simulink model "System_Modell"  (R2018a)
settings: Solver=FixedStepAuto  StartTime=0.0  StopTime=inf  FixedStep=1/f  RelTol=1e-3
values from neighbouring files (symbols this model uses):
  f = 10000    [System_Init.m]
(part 1 of 8)
settings Model: Creator=lenovo  LastModifiedBy=lenovo

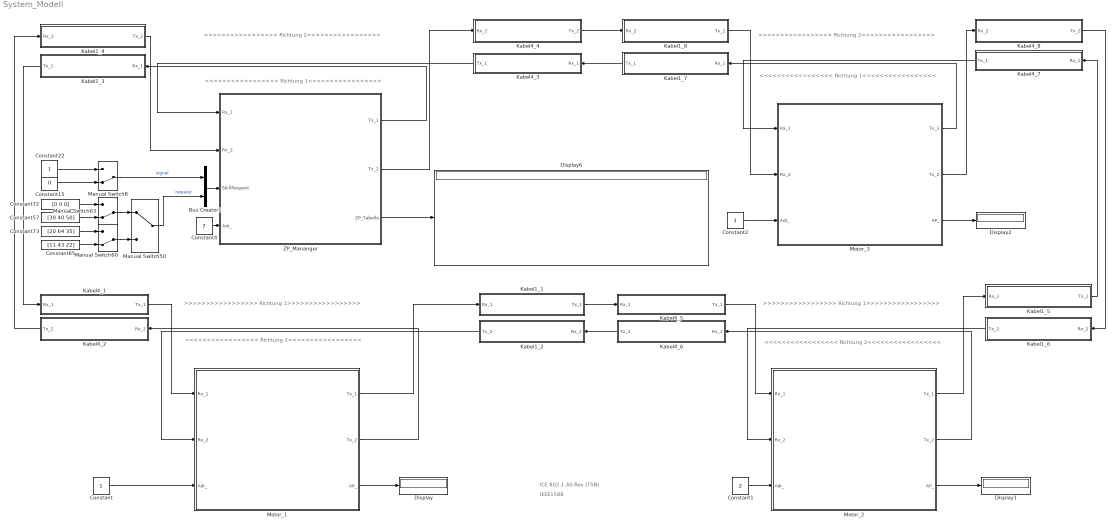
== system System_Modell ==
  note: >>>>>>>>>>>>>>>>> Richtung 1>>>>>>>>>>>>>>>>>
  note: <<<<<<<<<<<<<<<<< Richtung 2<<<<<<<<<<<<<<<<<
  note: ICE 802.1 AS-Rev (TSN)
  note: IEEE1588
  note: >>>>>>>>>>>>>>>>> Richtung 2>>>>>>>>>>>>>>>>>
  note: <<<<<<<<<<<<<<<<< Richtung 1<<<<<<<<<<<<<<<<<
  note: >>>>>>>>>>>>>>>>> Richtung 2>>>>>>>>>>>>>>>>>
  note: <<<<<<<<<<<<<<<<< Richtung 1<<<<<<<<<<<<<<<<<
  note: >>>>>>>>>>>>>>>>> Richtung 1>>>>>>>>>>>>>>>>>
  note: <<<<<<<<<<<<<<<<< Richtung 2<<<<<<<<<<<<<<<<<
  Bus Creator1 : BusCreator  Inputs=2
  Constant : Constant  OutDataTypeStr=double
  Constant1 : Constant  Value=2  OutDataTypeStr=double
  Constant15 : Constant  Value=0  OutDataTypeStr=boolean
  Constant2 : Constant  Value=3  OutDataTypeStr=double
  Constant22 : Constant  OutDataTypeStr=boolean
  Constant4 : Constant  Value=7  OutDataTypeStr=double
  Constant57 : Constant  Value=[30 40 50]
  Constant65 : Constant  Value=[11 43 22]
  Constant72 : Constant  Value=[0 0 0]
  Constant73 : Constant  Value=[20 64 35]
  Display{,1..2,6} (4 alike) : Display
  Kabel1_1 : Subsystem  TreatAsAtomicUnit=on
  Kabel1_2 : Subsystem  TreatAsAtomicUnit=on
  Kabel1_3 : Subsystem  TreatAsAtomicUnit=on
  Kabel1_4 : Subsystem  TreatAsAtomicUnit=on
  Kabel1_5 : Subsystem  TreatAsAtomicUnit=on
  Kabel1_6 : Subsystem  TreatAsAtomicUnit=on
  Kabel1_7 : Subsystem  TreatAsAtomicUnit=on
  Kabel1_8 : Subsystem  TreatAsAtomicUnit=on
  Kabel4_1 : Subsystem  TreatAsAtomicUnit=on
  Kabel4_2 : Subsystem  TreatAsAtomicUnit=on
  Kabel4_3 : Subsystem  TreatAsAtomicUnit=on
  Kabel4_4 : Subsystem  TreatAsAtomicUnit=on
  Kabel4_5 : Subsystem  TreatAsAtomicUnit=on
  Kabel4_6 : Subsystem  TreatAsAtomicUnit=on
  Kabel4_7 : Subsystem  TreatAsAtomicUnit=on
  Kabel4_8 : Subsystem  TreatAsAtomicUnit=on
  Manual Switch50 : ManualSwitch
  Manual Switch60 : ManualSwitch  CurrentSetting=0
  Manual Switch63 : ManualSwitch  CurrentSetting=0
  Manual Switch8 : ManualSwitch  CurrentSetting=0
  Motor_1 : Subsystem
  Motor_2 : Subsystem
  Motor_3 : Subsystem
  ZP_Mananger : Subsystem
  wires:
  Motor_1/2(Tx_2) -> Kabel4_2/1(Rx_2)
  Motor_1/3(AP_) -> Display/1
  Constant/1 -> Motor_1/3(Adr_)
  Kabel1_2/1(Tx_2) -> Motor_1/2(Rx_2)
  Kabel4_1/1(Tx_1) -> Motor_1/1(Rx_1)
  Constant22/1 -> Manual Switch8/1
  ZP_Mananger/3(ZP_Tabelle) -> Display6/1
  Constant65/1 -> Manual Switch60/2
  Constant15/1 -> Manual Switch8/2
  Manual Switch50/1 -> Bus Creator1/2  "request"
  ZP_Mananger/1(Tx_1) -> Kabel1_3/1(Rx_1)
  Bus Creator1/1 -> ZP_Mananger/3(SkillRequest)
  Manual Switch8/1 -> Bus Creator1/1  "signal"
  Kabel4_3/1(Tx_1) -> ZP_Mananger/1(Rx_1)
  Kabel1_4/1(Tx_2) -> ZP_Mananger/2(Rx_2)
  Constant72/1 -> Manual Switch63/1
  Manual Switch63/1 -> Manual Switch50/1
  Constant4/1 -> ZP_Mananger/4(Adr_)
  Constant57/1 -> Manual Switch63/2
  ZP_Mananger/2(Tx_2) -> Kabel4_4/1(Rx_2)
  Manual Switch60/1 -> Manual Switch50/2
  Constant73/1 -> Manual Switch60/1
  Kabel4_5/1(Tx_1) -> Motor_2/1(Rx_1)
  Kabel1_6/1(Tx_2) -> Motor_2/2(Rx_2)
  Constant1/1 -> Motor_2/3(Adr_)
  Motor_2/1(Tx_1) -> Kabel1_5/1(Rx_1)
  Motor_2/3(AP_) -> Display1/1
  Motor_2/2(Tx_2) -> Kabel4_6/1(Rx_2)
  Kabel4_6/1(Tx_2) -> Kabel1_2/1(Rx_2)
  Kabel1_1/1(Tx_1) -> Kabel4_5/1(Rx_1)
  Kabel4_7/1(Tx_1) -> Motor_3/1(Rx_1)
  Kabel1_8/1(Tx_2) -> Motor_3/2(Rx_2)
  Constant2/1 -> Motor_3/3(Adr_)
  Motor_3/1(Tx_1) -> Kabel1_7/1(Rx_1)
  Motor_3/3(AP_) -> Display2/1
  Motor_3/2(Tx_2) -> Kabel4_8/1(Rx_2)
  Kabel4_4/1(Tx_2) -> Kabel1_8/1(Rx_2)
  Kabel1_7/1(Tx_1) -> Kabel4_3/1(Rx_1)
  Kabel4_2/1(Tx_2) -> Kabel1_4/1(Rx_2)
  Kabel1_3/1(Tx_1) -> Kabel4_1/1(Rx_1)
  Kabel1_5/1(Tx_1) -> Kabel4_7/1(Rx_1)
  Kabel4_8/1(Tx_2) -> Kabel1_6/1(Rx_2)
  Motor_1/1(Tx_1) -> Kabel1_1/1(Rx_1)

== system System_Modell/Kabel1_1 ==
  In Bus Element : Inport  PortName=Rx_1  Element=signal
  In Bus Element1 : Inport  PortName=Rx_1  Element=data
  Delay1 : Delay  DelayLength=5
  Delay2 : Delay  DelayLength=5
  Out Bus Element : Outport  PortName=Tx_1  Element=signal
  Out Bus Element1 : Outport  PortName=Tx_1  Element=data
  wires:
  In Bus Element/1 -> Delay1/1
  Delay1/1 -> Out Bus Element/1
  In Bus Element1/1 -> Delay2/1
  Delay2/1 -> Out Bus Element1/1

== system System_Modell/Kabel1_2 ==
  In Bus Element : Inport  PortName=Rx_2  Element=signal
  In Bus Element1 : Inport  PortName=Rx_2  Element=data
  Delay1 : Delay  DelayLength=5
  Delay2 : Delay  DelayLength=5
  Out Bus Element : Outport  PortName=Tx_2  Element=signal
  Out Bus Element1 : Outport  PortName=Tx_2  Element=data
  wires:
  In Bus Element/1 -> Delay1/1
  Delay1/1 -> Out Bus Element/1
  In Bus Element1/1 -> Delay2/1
  Delay2/1 -> Out Bus Element1/1

== system System_Modell/Kabel1_3 ==
  In Bus Element : Inport  PortName=Rx_1  Element=signal
  In Bus Element1 : Inport  PortName=Rx_1  Element=data
  Delay1 : Delay  DelayLength=5
  Delay2 : Delay  DelayLength=5
  Telegramm_Stethoskop : MATLAB Function  TreatAsAtomicUnit=on
  Out Bus Element : Outport  PortName=Tx_1  Element=signal
  Out Bus Element1 : Outport  PortName=Tx_1  Element=data
  wires:
  Delay2/1 -> Out Bus Element1/1
  Delay1/1 -> Out Bus Element/1
  In Bus Element/1 -> Delay1/1
  In Bus Element1/1 -> Delay2/1

== system System_Modell/Kabel1_4 ==
  In Bus Element : Inport  PortName=Rx_2  Element=signal
  In Bus Element1 : Inport  PortName=Rx_2  Element=data
  Delay1 : Delay  DelayLength=5
  Delay2 : Delay  DelayLength=5
  Out Bus Element : Outport  PortName=Tx_2  Element=signal
  Out Bus Element1 : Outport  PortName=Tx_2  Element=data
  wires:
  In Bus Element/1 -> Delay1/1
  Delay1/1 -> Out Bus Element/1
  In Bus Element1/1 -> Delay2/1
  Delay2/1 -> Out Bus Element1/1

== system System_Modell/Kabel1_5 ==
  In Bus Element : Inport  PortName=Rx_1  Element=signal
  In Bus Element1 : Inport  PortName=Rx_1  Element=data
  Delay1 : Delay  DelayLength=5
  Delay2 : Delay  DelayLength=5
  Out Bus Element : Outport  PortName=Tx_1  Element=signal
  Out Bus Element1 : Outport  PortName=Tx_1  Element=data
  wires:
  In Bus Element/1 -> Delay1/1
  Delay1/1 -> Out Bus Element/1
  In Bus Element1/1 -> Delay2/1
  Delay2/1 -> Out Bus Element1/1

== system System_Modell/Kabel1_6 ==
  In Bus Element : Inport  PortName=Rx_2  Element=signal
  In Bus Element1 : Inport  PortName=Rx_2  Element=data
  Delay1 : Delay  DelayLength=5
  Delay2 : Delay  DelayLength=5
  Out Bus Element : Outport  PortName=Tx_2  Element=signal
  Out Bus Element1 : Outport  PortName=Tx_2  Element=data
  wires:
  In Bus Element/1 -> Delay1/1
  Delay1/1 -> Out Bus Element/1
  In Bus Element1/1 -> Delay2/1
  Delay2/1 -> Out Bus Element1/1

== system System_Modell/Kabel1_7 ==
  In Bus Element : Inport  PortName=Rx_1  Element=signal
  In Bus Element1 : Inport  PortName=Rx_1  Element=data
  Delay1 : Delay  DelayLength=10
  Delay2 : Delay  DelayLength=10
  Out Bus Element : Outport  PortName=Tx_1  Element=signal
  Out Bus Element1 : Outport  PortName=Tx_1  Element=data
  wires:
  In Bus Element/1 -> Delay1/1
  Delay1/1 -> Out Bus Element/1
  In Bus Element1/1 -> Delay2/1
  Delay2/1 -> Out Bus Element1/1

== system System_Modell/Kabel1_8 ==
  In Bus Element : Inport  PortName=Rx_2  Element=signal
  In Bus Element1 : Inport  PortName=Rx_2  Element=data
  Delay1 : Delay  DelayLength=5
  Delay2 : Delay  DelayLength=5
  Out Bus Element : Outport  PortName=Tx_2  Element=signal
  Out Bus Element1 : Outport  PortName=Tx_2  Element=data
  wires:
  In Bus Element/1 -> Delay1/1
  Delay1/1 -> Out Bus Element/1
  In Bus Element1/1 -> Delay2/1
  Delay2/1 -> Out Bus Element1/1

== system System_Modell/Kabel4_1 ==
  In Bus Element : Inport  PortName=Rx_1  Element=signal
  In Bus Element1 : Inport  PortName=Rx_1  Element=data
  Delay1 : Delay  DelayLength=5
  Delay2 : Delay  DelayLength=5
  Out Bus Element : Outport  PortName=Tx_1  Element=signal
  Out Bus Element1 : Outport  PortName=Tx_1  Element=data
  wires:
  Delay1/1 -> Out Bus Element/1
  Delay2/1 -> Out Bus Element1/1
  In Bus Element/1 -> Delay1/1
  In Bus Element1/1 -> Delay2/1

== system System_Modell/Kabel4_2 ==
  In Bus Element : Inport  PortName=Rx_2  Element=signal
  In Bus Element1 : Inport  PortName=Rx_2  Element=data
  Delay1 : Delay  DelayLength=5
  Delay2 : Delay  DelayLength=5
  Out Bus Element : Outport  PortName=Tx_2  Element=signal
  Out Bus Element1 : Outport  PortName=Tx_2  Element=data
  wires:
  In Bus Element/1 -> Delay1/1
  Delay1/1 -> Out Bus Element/1
  In Bus Element1/1 -> Delay2/1
  Delay2/1 -> Out Bus Element1/1

== system System_Modell/Kabel4_3 ==
  In Bus Element : Inport  PortName=Rx_1  Element=signal
  In Bus Element1 : Inport  PortName=Rx_1  Element=data
  Delay1 : Delay  DelayLength=5
  Delay2 : Delay  DelayLength=5
  Out Bus Element : Outport  PortName=Tx_1  Element=signal
  Out Bus Element1 : Outport  PortName=Tx_1  Element=data
  wires:
  Delay1/1 -> Out Bus Element/1
  Delay2/1 -> Out Bus Element1/1
  In Bus Element/1 -> Delay1/1
  In Bus Element1/1 -> Delay2/1

== system System_Modell/Kabel4_4 ==
  In Bus Element : Inport  PortName=Rx_2  Element=signal
  In Bus Element1 : Inport  PortName=Rx_2  Element=data
  Delay1 : Delay  DelayLength=5
  Delay2 : Delay  DelayLength=5
  Out Bus Element : Outport  PortName=Tx_2  Element=signal
  Out Bus Element1 : Outport  PortName=Tx_2  Element=data
  wires:
  In Bus Element/1 -> Delay1/1
  Delay1/1 -> Out Bus Element/1
  In Bus Element1/1 -> Delay2/1
  Delay2/1 -> Out Bus Element1/1

== system System_Modell/Kabel4_5 ==
  In Bus Element : Inport  PortName=Rx_1  Element=signal
  In Bus Element1 : Inport  PortName=Rx_1  Element=data
  Delay1 : Delay  DelayLength=5
  Delay2 : Delay  DelayLength=5
  Out Bus Element : Outport  PortName=Tx_1  Element=signal
  Out Bus Element1 : Outport  PortName=Tx_1  Element=data
  wires:
  In Bus Element/1 -> Delay1/1
  Delay1/1 -> Out Bus Element/1
  In Bus Element1/1 -> Delay2/1
  Delay2/1 -> Out Bus Element1/1

== system System_Modell/Kabel4_6 ==
  In Bus Element : Inport  PortName=Rx_2  Element=signal
  In Bus Element1 : Inport  PortName=Rx_2  Element=data
  Delay1 : Delay  DelayLength=5
  Delay2 : Delay  DelayLength=5
  Out Bus Element : Outport  PortName=Tx_2  Element=signal
  Out Bus Element1 : Outport  PortName=Tx_2  Element=data
  wires:
  In Bus Element/1 -> Delay1/1
  Delay1/1 -> Out Bus Element/1
  In Bus Element1/1 -> Delay2/1
  Delay2/1 -> Out Bus Element1/1

== system System_Modell/Kabel4_7 ==
  In Bus Element : Inport  PortName=Rx_1  Element=signal
  In Bus Element1 : Inport  PortName=Rx_1  Element=data
  Delay1 : Delay  DelayLength=5
  Delay2 : Delay  DelayLength=5
  Out Bus Element : Outport  PortName=Tx_1  Element=signal
  Out Bus Element1 : Outport  PortName=Tx_1  Element=data
  wires:
  In Bus Element/1 -> Delay1/1
  Delay1/1 -> Out Bus Element/1
  In Bus Element1/1 -> Delay2/1
  Delay2/1 -> Out Bus Element1/1

== system System_Modell/Kabel4_8 ==
  In Bus Element : Inport  PortName=Rx_2  Element=signal
  In Bus Element1 : Inport  PortName=Rx_2  Element=data
  Delay1 : Delay  DelayLength=5
  Delay2 : Delay  DelayLength=5
  Out Bus Element : Outport  PortName=Tx_2  Element=signal
  Out Bus Element1 : Outport  PortName=Tx_2  Element=data
  wires:
  In Bus Element/1 -> Delay1/1
  Delay1/1 -> Out Bus Element/1
  In Bus Element1/1 -> Delay2/1
  Delay2/1 -> Out Bus Element1/1

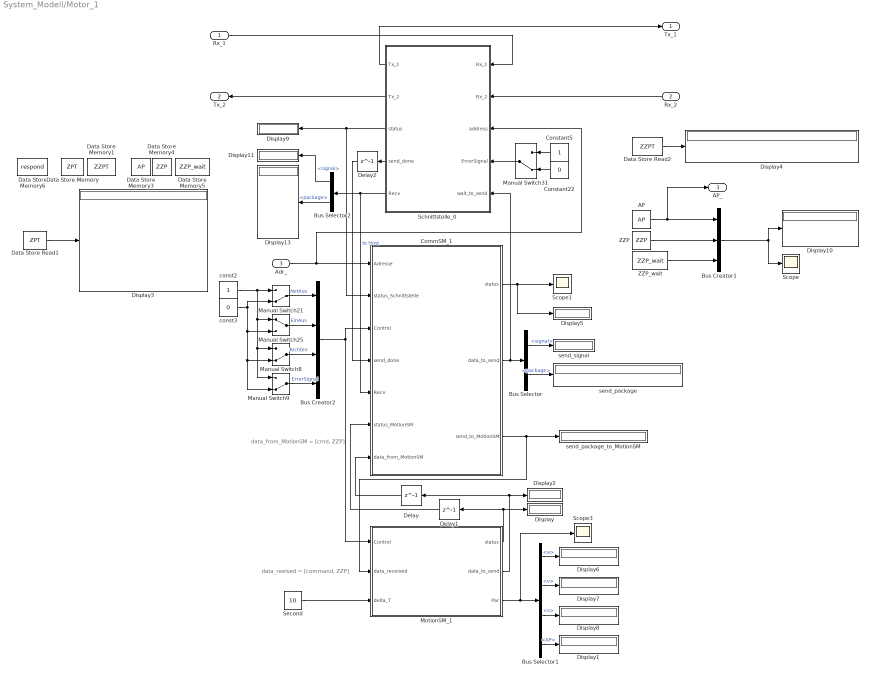
== system System_Modell/Motor_1 ==
  note: data_reeived = [command, ZZP]
  note: data_from_MotionSM = [cmd, ZZP]
  Rx_1 : Inport
  Rx_2 : Inport  Port=2
  Adr_ : Inport  Port=3
  AP : DataStoreRead  DataStoreName=AP
  Bus Creator1 : BusCreator  Inputs=3
  Bus Creator2 : BusCreator  Inputs=4
  Bus Selector : BusSelector  OutputSignals=signal,package
  Bus Selector1 : BusSelector  OutputSignals=a,v,s,AP
  Bus Selector2 : BusSelector  OutputSignals=signal,package
  CommSM_1 : Subsystem
  Constant22 : Constant  Value=0  OutDataTypeStr=boolean
  Constant5 : Constant  OutDataTypeStr=boolean
  Data Store Memory : DataStoreMemory  DataStoreName=ZPT  ReadBeforeWriteMsg=warning  WriteAfterWriteMsg=warning  WriteAfterReadMsg=warning  InitialValue=zeros(10,3)  VectorParams1D=off  ShowAdditionalParam=off  OutDataTypeStr=double  Dimensions=[10,3]
  Data Store Memory1 : DataStoreMemory  DataStoreName=ZZPT  ReadBeforeWriteMsg=warning  WriteAfterWriteMsg=warning  WriteAfterReadMsg=warning  InitialValue=zeros(3,4)  VectorParams1D=off  ShowAdditionalParam=off  OutDataTypeStr=double  Dimensions=[3,4]
  Data Store Memory3 : DataStoreMemory  DataStoreName=AP  ReadBeforeWriteMsg=warning  WriteAfterWriteMsg=warning  WriteAfterReadMsg=warning  ShowAdditionalParam=off  OutMin=[0]  OutMax=[100]  OutDataTypeStr=double  Dimensions=1
  Data Store Memory4 : DataStoreMemory  DataStoreName=ZZP  ReadBeforeWriteMsg=warning  WriteAfterWriteMsg=warning  WriteAfterReadMsg=warning  ShowAdditionalParam=off  OutDataTypeStr=double  Dimensions=1
  Data Store Memory5 : DataStoreMemory  DataStoreName=ZZP_wait  ReadBeforeWriteMsg=warning  WriteAfterWriteMsg=warning  WriteAfterReadMsg=warning  ShowAdditionalParam=off  OutDataTypeStr=double  Dimensions=1
  Data Store Memory6 : DataStoreMemory  DataStoreName=respond  ReadBeforeWriteMsg=warning  WriteAfterWriteMsg=warning  WriteAfterReadMsg=warning  InitialValue=false  ShowAdditionalParam=off  OutDataTypeStr=boolean  Dimensions=1
  Data Store Read1 : DataStoreRead  DataStoreName=ZPT
  Data Store Read2 : DataStoreRead  DataStoreName=ZZPT
  Delay : Delay  DelayLength=1
  Delay1 : Delay  DelayLength=1
  Delay2 : Delay  DelayLength=1
  Display{,1..11,13} (13 alike) : Display
      Display1 settings: Format=decimal (Stored Integer)
      Display10 settings: Format=decimal (Stored Integer)
      Display13 settings: Decimation=7
      Display8 settings: Format=decimal (Stored Integer)
  Manual Switch{8..9,21,31} (4 alike) : ManualSwitch  CurrentSetting=0
  Manual Switch25 : ManualSwitch
  MotionSM_1 : Subsystem
  Schnittstelle_0 : Subsystem
  Scope : Scope
  Scope1 : Scope
  Scope3 : Scope
  Second : Constant  Value=10
  ZZP : DataStoreRead  DataStoreName=ZZP
  ZZP_wait : DataStoreRead  DataStoreName=ZZP_wait
  const2 : Constant  OutDataTypeStr=boolean
  const3 : Constant  Value=0  OutDataTypeStr=boolean
  send_package : Display
  send_package_to_MotionSM : Display
  send_signal : Display
  Tx_1 : Outport
  Tx_2 : Outport  Port=2
  AP_ : Outport  Port=3
  wires:
  Bus Creator2/1 -> MotionSM_1/1(Control), CommSM_1/3(Control)
  MotionSM_1/2(data_to_send) -> Delay/1, Display2/1
  Constant22/1 -> Manual Switch31/2
  Bus Selector2/2 -> Display13/1  "<package>"
  CommSM_1/3(send_to_MotionSM) -> send_package_to_MotionSM/1, MotionSM_1/2(data_received)
  MotionSM_1/3(Par) -> Scope3/1, Bus Selector1/1
  Data Store Read1/1 -> Display3/1
  MotionSM_1/1(status) -> Display/1, Delay1/1
  Manual Switch25/1 -> Bus Creator2/2  "EinAus"
  Delay/1 -> CommSM_1/7(data_from_MotionSM)
  const2/1 -> Manual Switch9/1, Manual Switch8/1, Manual Switch25/1, Manual Switch21/1
  Manual Switch21/1 -> Bus Creator2/1  "NotAus"
  CommSM_1/1(status) -> Display5/1, Scope1/1
  Constant5/1 -> Manual Switch31/1
  Bus Creator1/1 -> Display10/1, Scope/1
  Delay1/1 -> CommSM_1/6(status_MotionSM)
  CommSM_1/2(data_to_send) -> Bus Selector/1, Schnittstelle_0/5(wait_to_send)
  const3/1 -> Manual Switch21/2, Manual Switch9/2, Manual Switch8/2, Manual Switch25/2
  Second/1 -> MotionSM_1/3(delta_T)
  AP/1 -> AP_/1, Bus Creator1/1
  Bus Selector1/4 -> Display1/1  "<AP>"
  Schnittstelle_0/5(Recv) -> CommSM_1/5(Recv), Bus Selector2/1  "to Host"
  Bus Selector/2 -> send_package/1  "<package>"
  Manual Switch31/1 -> Schnittstelle_0/4(ErrorSignal)
  Manual Switch8/1 -> Bus Creator2/3  "Richten"
  Bus Selector2/1 -> Display11/1  "<signal>"
  Bus Selector1/2 -> Display7/1  "<v>"
  Manual Switch9/1 -> Bus Creator2/4  "ErrorSignal"
  Rx_1/1 -> Schnittstelle_0/1(Rx_1)
  ZZP_wait/1 -> Bus Creator1/3
  ZZP/1 -> Bus Creator1/2
  Data Store Read2/1 -> Display4/1
  Bus Selector1/1 -> Display6/1  "<a>"
  Schnittstelle_0/3(status) -> Display9/1, CommSM_1/2(status_Schnittstelle)
  Bus Selector/1 -> send_signal/1  "<signal>"
  Bus Selector1/3 -> Display8/1  "<s>"
  Schnittstelle_0/2(Tx_2) -> Tx_2/1
  Rx_2/1 -> Schnittstelle_0/2(Rx_2)
  Schnittstelle_0/1(Tx_1) -> Tx_1/1
  Adr_/1 -> Schnittstelle_0/3(address), CommSM_1/1(Adresse)
  Delay2/1 -> CommSM_1/4(send_done)
  Schnittstelle_0/4(send_done) -> Delay2/1

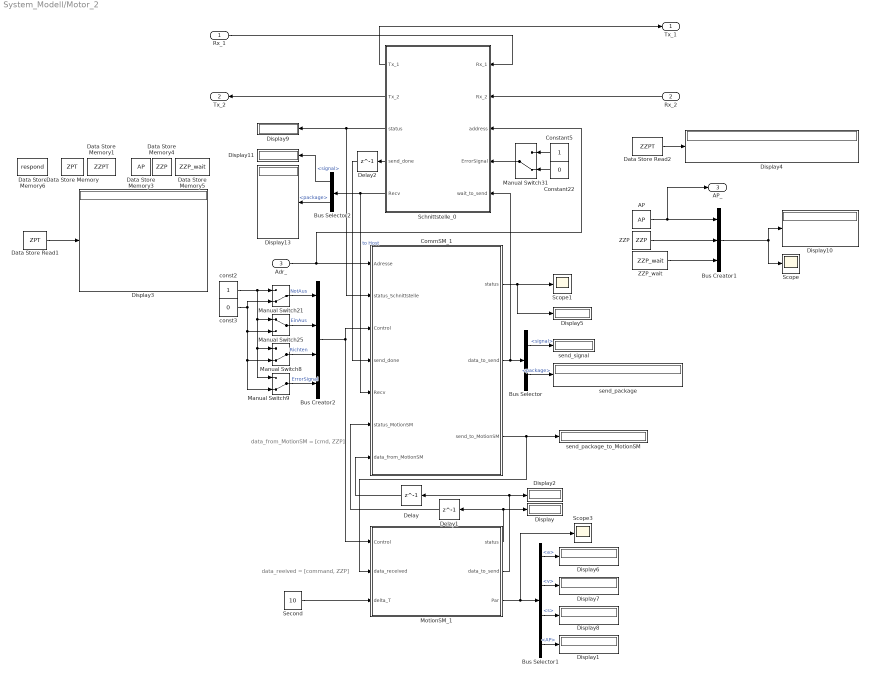
== system System_Modell/Motor_2 ==
  note: data_reeived = [command, ZZP]
  note: data_from_MotionSM = [cmd, ZZP]
  Rx_1 : Inport
  Rx_2 : Inport  Port=2
  Adr_ : Inport  Port=3
  AP : DataStoreRead  DataStoreName=AP
  Bus Creator1 : BusCreator  Inputs=3
  Bus Creator2 : BusCreator  Inputs=4
  Bus Selector : BusSelector  OutputSignals=signal,package
  Bus Selector1 : BusSelector  OutputSignals=a,v,s,AP
  Bus Selector2 : BusSelector  OutputSignals=signal,package
  CommSM_1 : Subsystem
  Constant22 : Constant  Value=0  OutDataTypeStr=boolean
  Constant5 : Constant  OutDataTypeStr=boolean
  Data Store Memory : DataStoreMemory  DataStoreName=ZPT  ReadBeforeWriteMsg=warning  WriteAfterWriteMsg=warning  WriteAfterReadMsg=warning  InitialValue=zeros(10,3)  VectorParams1D=off  ShowAdditionalParam=off  OutDataTypeStr=double  Dimensions=[10,3]
  Data Store Memory1 : DataStoreMemory  DataStoreName=ZZPT  ReadBeforeWriteMsg=warning  WriteAfterWriteMsg=warning  WriteAfterReadMsg=warning  InitialValue=zeros(3,4)  VectorParams1D=off  ShowAdditionalParam=off  OutDataTypeStr=double  Dimensions=[3,4]
  Data Store Memory3 : DataStoreMemory  DataStoreName=AP  ReadBeforeWriteMsg=warning  WriteAfterWriteMsg=warning  WriteAfterReadMsg=warning  ShowAdditionalParam=off  OutMin=[0]  OutMax=[100]  OutDataTypeStr=double  Dimensions=1
  Data Store Memory4 : DataStoreMemory  DataStoreName=ZZP  ReadBeforeWriteMsg=warning  WriteAfterWriteMsg=warning  WriteAfterReadMsg=warning  ShowAdditionalParam=off  OutDataTypeStr=double  Dimensions=1
  Data Store Memory5 : DataStoreMemory  DataStoreName=ZZP_wait  ReadBeforeWriteMsg=warning  WriteAfterWriteMsg=warning  WriteAfterReadMsg=warning  ShowAdditionalParam=off  OutDataTypeStr=double  Dimensions=1
  Data Store Memory6 : DataStoreMemory  DataStoreName=respond  ReadBeforeWriteMsg=warning  WriteAfterWriteMsg=warning  WriteAfterReadMsg=warning  InitialValue=false  ShowAdditionalParam=off  OutDataTypeStr=boolean  Dimensions=1
  Data Store Read1 : DataStoreRead  DataStoreName=ZPT
  Data Store Read2 : DataStoreRead  DataStoreName=ZZPT
  Delay : Delay  DelayLength=1
  Delay1 : Delay  DelayLength=1
  Delay2 : Delay  DelayLength=1
  Display{,1..11,13} (13 alike) : Display
      Display1 settings: Format=decimal (Stored Integer)
      Display10 settings: Format=decimal (Stored Integer)
      Display13 settings: Decimation=7
      Display8 settings: Format=decimal (Stored Integer)
  Manual Switch{8..9,21,31} (4 alike) : ManualSwitch  CurrentSetting=0
  Manual Switch25 : ManualSwitch
  MotionSM_1 : Subsystem
  Schnittstelle_0 : Subsystem
  Scope : Scope
  Scope1 : Scope
  Scope3 : Scope
  Second : Constant  Value=10
  ZZP : DataStoreRead  DataStoreName=ZZP
  ZZP_wait : DataStoreRead  DataStoreName=ZZP_wait
  const2 : Constant  OutDataTypeStr=boolean
  const3 : Constant  Value=0  OutDataTypeStr=boolean
  send_package : Display
  send_package_to_MotionSM : Display
  send_signal : Display
  Tx_1 : Outport
  Tx_2 : Outport  Port=2
  AP_ : Outport  Port=3
  wires:
  Bus Creator2/1 -> MotionSM_1/1(Control), CommSM_1/3(Control)
  MotionSM_1/2(data_to_send) -> Delay/1, Display2/1
  Constant22/1 -> Manual Switch31/2
  Bus Selector2/2 -> Display13/1  "<package>"
  CommSM_1/3(send_to_MotionSM) -> send_package_to_MotionSM/1, MotionSM_1/2(data_received)
  MotionSM_1/3(Par) -> Scope3/1, Bus Selector1/1
  Data Store Read1/1 -> Display3/1
  MotionSM_1/1(status) -> Display/1, Delay1/1
  Manual Switch25/1 -> Bus Creator2/2  "EinAus"
  Delay/1 -> CommSM_1/7(data_from_MotionSM)
  const2/1 -> Manual Switch9/1, Manual Switch8/1, Manual Switch25/1, Manual Switch21/1
  Manual Switch21/1 -> Bus Creator2/1  "NotAus"
  CommSM_1/1(status) -> Display5/1, Scope1/1
  Constant5/1 -> Manual Switch31/1
  Bus Creator1/1 -> Display10/1, Scope/1
  Delay1/1 -> CommSM_1/6(status_MotionSM)
  CommSM_1/2(data_to_send) -> Bus Selector/1, Schnittstelle_0/5(wait_to_send)
  const3/1 -> Manual Switch21/2, Manual Switch9/2, Manual Switch8/2, Manual Switch25/2
  Second/1 -> MotionSM_1/3(delta_T)
  AP/1 -> AP_/1, Bus Creator1/1
  Bus Selector1/4 -> Display1/1  "<AP>"
  Schnittstelle_0/5(Recv) -> CommSM_1/5(Recv), Bus Selector2/1  "to Host"
  Bus Selector/2 -> send_package/1  "<package>"
  Manual Switch31/1 -> Schnittstelle_0/4(ErrorSignal)
  Manual Switch8/1 -> Bus Creator2/3  "Richten"
  Bus Selector2/1 -> Display11/1  "<signal>"
  Bus Selector1/2 -> Display7/1  "<v>"
  Manual Switch9/1 -> Bus Creator2/4  "ErrorSignal"
  Rx_1/1 -> Schnittstelle_0/1(Rx_1)
  ZZP_wait/1 -> Bus Creator1/3
  ZZP/1 -> Bus Creator1/2
  Data Store Read2/1 -> Display4/1
  Bus Selector1/1 -> Display6/1  "<a>"
  Schnittstelle_0/3(status) -> Display9/1, CommSM_1/2(status_Schnittstelle)
  Bus Selector/1 -> send_signal/1  "<signal>"
  Bus Selector1/3 -> Display8/1  "<s>"
  Schnittstelle_0/2(Tx_2) -> Tx_2/1
  Rx_2/1 -> Schnittstelle_0/2(Rx_2)
  Schnittstelle_0/1(Tx_1) -> Tx_1/1
  Adr_/1 -> Schnittstelle_0/3(address), CommSM_1/1(Adresse)
  Delay2/1 -> CommSM_1/4(send_done)
  Schnittstelle_0/4(send_done) -> Delay2/1

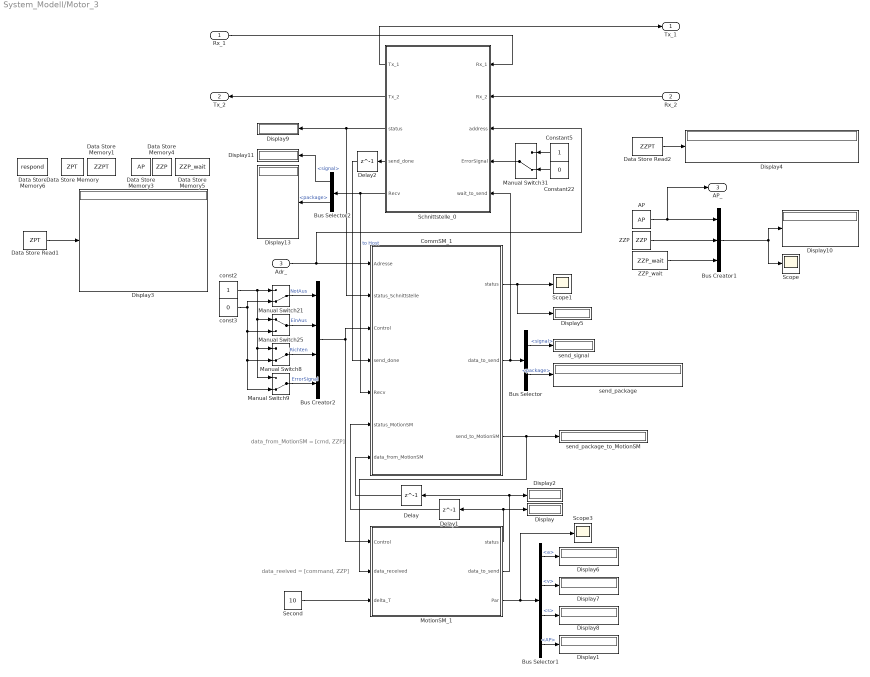
== system System_Modell/Motor_3 ==
  note: data_reeived = [command, ZZP]
  note: data_from_MotionSM = [cmd, ZZP]
  Rx_1 : Inport
  Rx_2 : Inport  Port=2
  Adr_ : Inport  Port=3
  AP : DataStoreRead  DataStoreName=AP
  Bus Creator1 : BusCreator  Inputs=3
  Bus Creator2 : BusCreator  Inputs=4
  Bus Selector : BusSelector  OutputSignals=signal,package
  Bus Selector1 : BusSelector  OutputSignals=a,v,s,AP
  Bus Selector2 : BusSelector  OutputSignals=signal,package
  CommSM_1 : Subsystem
  Constant22 : Constant  Value=0  OutDataTypeStr=boolean
  Constant5 : Constant  OutDataTypeStr=boolean
  Data Store Memory : DataStoreMemory  DataStoreName=ZPT  ReadBeforeWriteMsg=warning  WriteAfterWriteMsg=warning  WriteAfterReadMsg=warning  InitialValue=zeros(10,3)  VectorParams1D=off  ShowAdditionalParam=off  OutDataTypeStr=double  Dimensions=[10,3]
  Data Store Memory1 : DataStoreMemory  DataStoreName=ZZPT  ReadBeforeWriteMsg=warning  WriteAfterWriteMsg=warning  WriteAfterReadMsg=warning  InitialValue=zeros(3,4)  VectorParams1D=off  ShowAdditionalParam=off  OutDataTypeStr=double  Dimensions=[3,4]
  Data Store Memory3 : DataStoreMemory  DataStoreName=AP  ReadBeforeWriteMsg=warning  WriteAfterWriteMsg=warning  WriteAfterReadMsg=warning  ShowAdditionalParam=off  OutMin=[0]  OutMax=[100]  OutDataTypeStr=double  Dimensions=1
  Data Store Memory4 : DataStoreMemory  DataStoreName=ZZP  ReadBeforeWriteMsg=warning  WriteAfterWriteMsg=warning  WriteAfterReadMsg=warning  ShowAdditionalParam=off  OutDataTypeStr=double  Dimensions=1
  Data Store Memory5 : DataStoreMemory  DataStoreName=ZZP_wait  ReadBeforeWriteMsg=warning  WriteAfterWriteMsg=warning  WriteAfterReadMsg=warning  ShowAdditionalParam=off  OutDataTypeStr=double  Dimensions=1
  Data Store Memory6 : DataStoreMemory  DataStoreName=respond  ReadBeforeWriteMsg=warning  WriteAfterWriteMsg=warning  WriteAfterReadMsg=warning  InitialValue=false  ShowAdditionalParam=off  OutDataTypeStr=boolean  Dimensions=1
  Data Store Read1 : DataStoreRead  DataStoreName=ZPT
  Data Store Read2 : DataStoreRead  DataStoreName=ZZPT
  Delay : Delay  DelayLength=1
  Delay1 : Delay  DelayLength=1
  Delay2 : Delay  DelayLength=1
  Display{,1..11,13} (13 alike) : Display
      Display1 settings: Format=decimal (Stored Integer)
      Display10 settings: Format=decimal (Stored Integer)
      Display13 settings: Decimation=7
      Display8 settings: Format=decimal (Stored Integer)
  Manual Switch{8..9,21,31} (4 alike) : ManualSwitch  CurrentSetting=0
  Manual Switch25 : ManualSwitch
  MotionSM_1 : Subsystem
  Schnittstelle_0 : Subsystem
  Scope : Scope
  Scope1 : Scope
  Scope3 : Scope
  Second : Constant  Value=10
  ZZP : DataStoreRead  DataStoreName=ZZP
  ZZP_wait : DataStoreRead  DataStoreName=ZZP_wait
  const2 : Constant  OutDataTypeStr=boolean
  const3 : Constant  Value=0  OutDataTypeStr=boolean
  send_package : Display
  send_package_to_MotionSM : Display
  send_signal : Display
  Tx_1 : Outport
  Tx_2 : Outport  Port=2
  AP_ : Outport  Port=3
  wires:
  Bus Creator2/1 -> MotionSM_1/1(Control), CommSM_1/3(Control)
  MotionSM_1/2(data_to_send) -> Delay/1, Display2/1
  Constant22/1 -> Manual Switch31/2
  Bus Selector2/2 -> Display13/1  "<package>"
  CommSM_1/3(send_to_MotionSM) -> send_package_to_MotionSM/1, MotionSM_1/2(data_received)
  MotionSM_1/3(Par) -> Scope3/1, Bus Selector1/1
  Data Store Read1/1 -> Display3/1
  MotionSM_1/1(status) -> Display/1, Delay1/1
  Manual Switch25/1 -> Bus Creator2/2  "EinAus"
  Delay/1 -> CommSM_1/7(data_from_MotionSM)
  const2/1 -> Manual Switch9/1, Manual Switch8/1, Manual Switch25/1, Manual Switch21/1
  Manual Switch21/1 -> Bus Creator2/1  "NotAus"
  CommSM_1/1(status) -> Display5/1, Scope1/1
  Constant5/1 -> Manual Switch31/1
  Bus Creator1/1 -> Display10/1, Scope/1
  Delay1/1 -> CommSM_1/6(status_MotionSM)
  CommSM_1/2(data_to_send) -> Bus Selector/1, Schnittstelle_0/5(wait_to_send)
  const3/1 -> Manual Switch21/2, Manual Switch9/2, Manual Switch8/2, Manual Switch25/2
  Second/1 -> MotionSM_1/3(delta_T)
  AP/1 -> AP_/1, Bus Creator1/1
  Bus Selector1/4 -> Display1/1  "<AP>"
  Schnittstelle_0/5(Recv) -> CommSM_1/5(Recv), Bus Selector2/1  "to Host"
  Bus Selector/2 -> send_package/1  "<package>"
  Manual Switch31/1 -> Schnittstelle_0/4(ErrorSignal)
  Manual Switch8/1 -> Bus Creator2/3  "Richten"
  Bus Selector2/1 -> Display11/1  "<signal>"
  Bus Selector1/2 -> Display7/1  "<v>"
  Manual Switch9/1 -> Bus Creator2/4  "ErrorSignal"
  Rx_1/1 -> Schnittstelle_0/1(Rx_1)
  ZZP_wait/1 -> Bus Creator1/3
  ZZP/1 -> Bus Creator1/2
  Data Store Read2/1 -> Display4/1
  Bus Selector1/1 -> Display6/1  "<a>"
  Schnittstelle_0/3(status) -> Display9/1, CommSM_1/2(status_Schnittstelle)
  Bus Selector/1 -> send_signal/1  "<signal>"
  Bus Selector1/3 -> Display8/1  "<s>"
  Schnittstelle_0/2(Tx_2) -> Tx_2/1
  Rx_2/1 -> Schnittstelle_0/2(Rx_2)
  Schnittstelle_0/1(Tx_1) -> Tx_1/1
  Adr_/1 -> Schnittstelle_0/3(address), CommSM_1/1(Adresse)
  Delay2/1 -> CommSM_1/4(send_done)
  Schnittstelle_0/4(send_done) -> Delay2/1

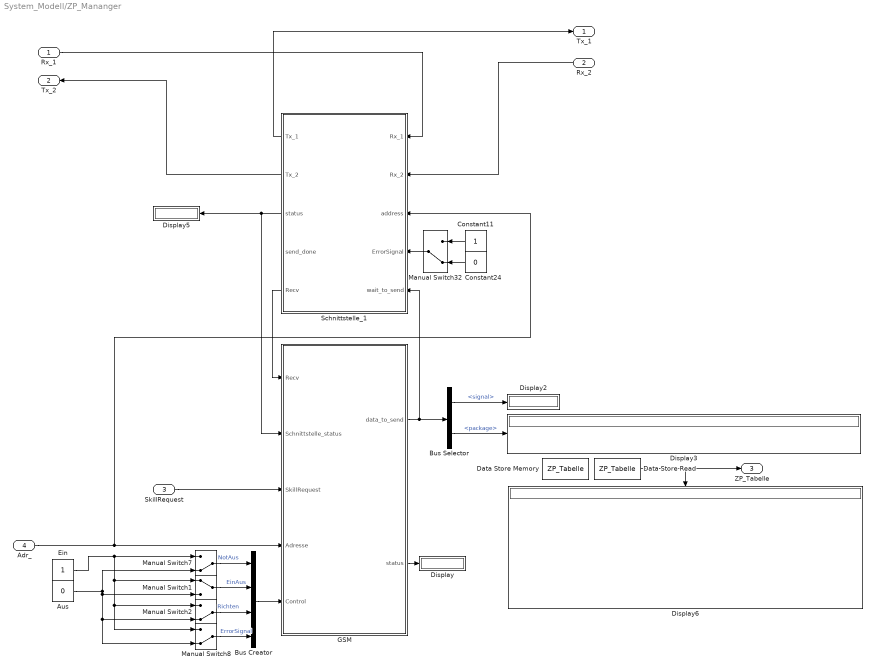
== system System_Modell/ZP_Mananger ==
  Rx_1 : Inport
  Rx_2 : Inport  Port=2
  SkillRequest : Inport  Port=3
  Adr_ : Inport  Port=4
  Aus : Constant  Value=0  OutDataTypeStr=boolean
  Bus Creator : BusCreator  Inputs=4
  Bus Selector : BusSelector  OutputSignals=signal,package
  Constant11 : Constant  OutDataTypeStr=boolean
  Constant24 : Constant  Value=0  OutDataTypeStr=boolean
  Data Store Memory : DataStoreMemory  DataStoreName=ZP_Tabelle  ReadBeforeWriteMsg=warning  WriteAfterWriteMsg=warning  WriteAfterReadMsg=warning  InitialValue=zeros(10,7)  ShowAdditionalParam=off  OutDataTypeStr=double  Dimensions=[10 7]
  Data Store Read : DataStoreRead  DataStoreName=ZP_Tabelle
  Display{,2..3,5..6} (5 alike) : Display
  Ein : Constant  OutDataTypeStr=boolean
  "GSM " : Subsystem
  Manual Switch1 : ManualSwitch
  Manual Switch{2,7..8,32} (4 alike) : ManualSwitch  CurrentSetting=0
  Schnittstelle_1 : Subsystem
  Tx_1 : Outport
  Tx_2 : Outport  Port=2
  ZP_Tabelle : Outport  Port=3
  wires:
  Bus Selector/1 -> Display2/1  "<signal>"
  Ein/1 -> Manual Switch7/1, Manual Switch1/1, Manual Switch2/1, Manual Switch8/1
  Data Store Read/1 -> ZP_Tabelle/1, Display6/1
  Schnittstelle_1/5(Recv) -> "GSM "/1(Recv)
  Aus/1 -> Manual Switch7/2, Manual Switch1/2, Manual Switch2/2, Manual Switch8/2
  Manual Switch32/1 -> Schnittstelle_1/4(ErrorSignal)
  Manual Switch1/1 -> Bus Creator/2  "EinAus"
  Manual Switch8/1 -> Bus Creator/4  "ErrorSignal"
  Bus Selector/2 -> Display3/1  "<package>"
  "GSM "/2(status) -> Display/1
  Schnittstelle_1/3(status) -> "GSM "/2(Schnittstelle_status), Display5/1
  Manual Switch2/1 -> Bus Creator/3  "Richten"
  "GSM "/1(data_to_send) -> Bus Selector/1, Schnittstelle_1/5(wait_to_send)
  Bus Creator/1 -> "GSM "/5(Control)
  Constant24/1 -> Manual Switch32/2
  Constant11/1 -> Manual Switch32/1
  Manual Switch7/1 -> Bus Creator/1  "NotAus"
  Schnittstelle_1/1(Tx_1) -> Tx_1/1
  Rx_1/1 -> Schnittstelle_1/1(Rx_1)
  Rx_2/1 -> Schnittstelle_1/2(Rx_2)
  Schnittstelle_1/2(Tx_2) -> Tx_2/1
  Adr_/1 -> Schnittstelle_1/3(address), "GSM "/4(Adresse)
  SkillRequest/1 -> "GSM "/3(SkillRequest)

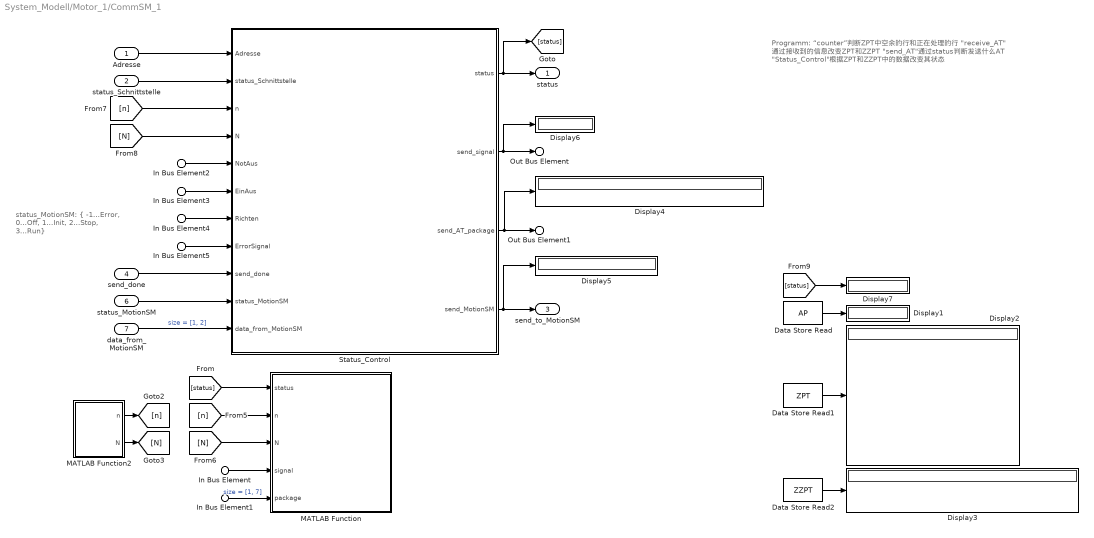
== system System_Modell/Motor_1/CommSM_1 ==
  note: Programm:
      | “counter”判断ZPT中空余的行和正在处理的行
      | "receive_AT" 通过接收到的信息改变ZPT和ZZPT
      | "send_AT"通过status判断发送什么AT
      | "Status_Control"根据ZPT和ZZPT中的数据改变其状态
  note: status_MotionSM: {
      | -1...Error,
      | 0...Off,
      | 1...Init,
      | 2...Stop,
      | 3...Run}
  Adresse : Inport  OutDataTypeStr=double  PortDimensions=1
  status_Schnittstelle : Inport  Port=2  OutDataTypeStr=double  PortDimensions=1
  In Bus Element2 : Inport  Port=3  PortName=Control  Element=NotAus
  In Bus Element3 : Inport  Port=3  PortName=Control  Element=EinAus
  In Bus Element4 : Inport  Port=3  PortName=Control  Element=Richten
  In Bus Element5 : Inport  Port=3  PortName=Control  Element=ErrorSignal
  send_done : Inport  Port=4
  In Bus Element : Inport  Port=5  PortName=Recv  Element=signal
  In Bus Element1 : Inport  Port=5  PortName=Recv  Element=package
  status_MotionSM : Inport  Port=6  OutDataTypeStr=double  PortDimensions=1
  data_from_MotionSM : Inport  Port=7  OutDataTypeStr=double  PortDimensions=2
  Data Store Read : DataStoreRead  DataStoreName=AP
  Data Store Read1 : DataStoreRead  DataStoreName=ZPT
  Data Store Read2 : DataStoreRead  DataStoreName=ZZPT
  Display{1..7} (7 alike) : Display
  MATLAB Function : MATLAB Function  TreatAsAtomicUnit=on
  MATLAB Function2 : MATLAB Function  TreatAsAtomicUnit=on
  Status_Control : Stateflow chart  TreatAsAtomicUnit=on
  status : Outport  OutDataTypeStr=double  PortDimensions=1
  Out Bus Element : Outport  Port=2  PortName=data_to_send  Element=signal
  Out Bus Element1 : Outport  Port=2  PortName=data_to_send  Element=package
  send_to_MotionSM : Outport  Port=3
  wires:
  In Bus Element2/1 -> Status_Control/5(NotAus)
  In Bus Element3/1 -> Status_Control/6(EinAus)
  In Bus Element4/1 -> Status_Control/7(Richten)
  In Bus Element5/1 -> Status_Control/8(ErrorSignal)
  status_Schnittstelle/1 -> Status_Control/2(status_Schnittstelle)
  In Bus Element/1 -> MATLAB Function/4(signal)
  In Bus Element1/1 -> MATLAB Function/5(package)  "size = [1, 7]"
  data_from_MotionSM/1 -> Status_Control/11(data_from_MotionSM)  "size = [1, 2]"
  status_MotionSM/1 -> Status_Control/10(status_MotionSM)
  Adresse/1 -> Status_Control/1(Adresse)
  Status_Control/1(status) -> [status], status/1
  Status_Control/3(send_AT_package) -> Out Bus Element1/1, Display4/1
  Status_Control/4(send_MotionSM) -> send_to_MotionSM/1, Display5/1
  Status_Control/2(send_signal) -> Out Bus Element/1, Display6/1
  Data Store Read/1 -> Display1/1
  Data Store Read1/1 -> Display2/1
  Data Store Read2/1 -> Display3/1
  [status] -> MATLAB Function/1(status)
  MATLAB Function2/1(n) -> [n]
  MATLAB Function2/2(N) -> [N]
  [N] -> MATLAB Function/3(N)
  [n] -> MATLAB Function/2(n)
  [n] -> Status_Control/3(n)
  [N] -> Status_Control/4(N)
  [status] -> Display7/1
  send_done/1 -> Status_Control/9(send_done)

== system System_Modell/Motor_1/MotionSM_1 ==
  note: parameter = [delta_T, a_max, v_max, s0]
  In Bus Element : Inport  PortName=Control  Element=NotAus
  In Bus Element1 : Inport  PortName=Control  Element=EinAus
  In Bus Element2 : Inport  PortName=Control  Element=Richten
  In Bus Element3 : Inport  PortName=Control  Element=ErrorSignal
  data_received : Inport  Port=2  OutDataTypeStr=double  PortDimensions=2
  delta_T : Inport  Port=3
  Bus Creator : BusCreator  Inputs=3
  Chart : Stateflow chart  TreatAsAtomicUnit=on
  Data Store Read : DataStoreRead  DataStoreName=AP
  Delay : Delay  DelayLength=1
  Delay1 : Delay  DelayLength=1
  Display{1..2,4..7} (6 alike) : Display
  MATLAB Function : MATLAB Function  TreatAsAtomicUnit=on
  Motor : Subsystem
  status : Outport
  data_to_send : Outport  Port=2  OutDataTypeStr=double  PortDimensions=2
  Out Bus Element : Outport  Port=3  PortName=Par  Element=a
  Out Bus Element1 : Outport  Port=3  PortName=Par  Element=v
  Out Bus Element2 : Outport  Port=3  PortName=Par  Element=s
  Out Bus Element3 : Outport  Port=3  PortName=Par  Element=AP
  wires:
  Chart/1(status) -> Motor/1(auto_control), Delay/1, Display1/1, status/1
  In Bus Element1/1 -> Chart/2(EinAus)
  In Bus Element/1 -> Chart/1(NotAus)
  In Bus Element2/1 -> Chart/3(Richten)
  In Bus Element3/1 -> Chart/4(ErrorSignal)
  Motor/1(status_Motor) -> Display4/1, Delay1/1
  data_received/1 -> MATLAB Function/2(data_received)
  Delay1/1 -> Chart/6(Motor_status)
  MATLAB Function/1(excute_signal) -> Display6/1, Chart/5(excute_signal)
  MATLAB Function/2(message_to_send) -> data_to_send/1, Display7/1  "size = [1, 2]"
  delta_T/1 -> Chart/7(delta_T)
  Motor/2(a) -> Bus Creator/3, Out Bus Element/1
  Motor/3(v) -> Bus Creator/2, Out Bus Element1/1
  Motor/4(s) -> Bus Creator/1, Out Bus Element2/1
  Chart/2(parameter) -> Motor/2(parameter), Display5/1
  Delay/1 -> MATLAB Function/1(status)
  Data Store Read/1 -> Out Bus Element3/1
  Bus Creator/1 -> Display2/1

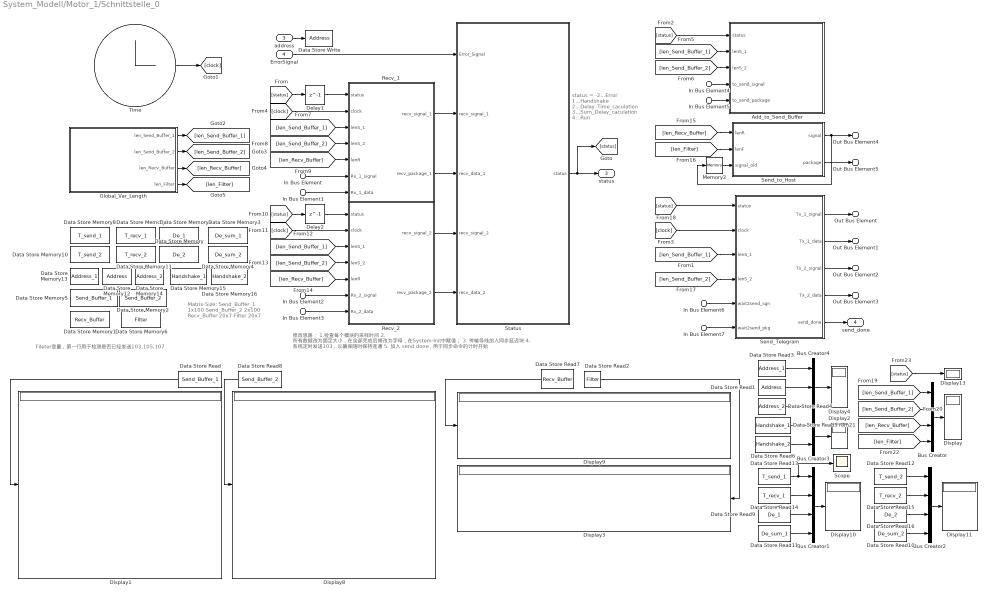
== system System_Modell/Motor_1/Schnittstelle_0 ==
  note: Fileter变量，第一行用于检测是否已经发送103,105,107
  note: 修改思路：
      | 1.检查每个模块的采样时间
      | 2. 所有数据改为固定大小，在全部完成后修改为字母，在System-Init中赋值；
      | 3. 传输导线加入同步延迟块
      | 4. 系统定时发送103，以确保随时保持连通
      | 5. 加入 send done，用于同步命令的计时开始
  note: status =
      | -2...Error
      |  1...Handshake
      |  2...Delay_Time_caculation
      |  3...Sum_Delay_caculation
      |  4...Run
  note: Matrix-Size:
      | Send_Buffer_1	1x100
      | Send_Buffer_2	2x100
      | Recv_Buffer		20x7
      | Filter			20x7
  In Bus Element : Inport  PortName=Rx_1  Element=signal
  In Bus Element1 : Inport  PortName=Rx_1  Element=data
  In Bus Element2 : Inport  Port=2  PortName=Rx_2  Element=signal
  In Bus Element3 : Inport  Port=2  PortName=Rx_2  Element=data
  address : Inport  Port=3
  ErrorSignal : Inport  Port=4
  In Bus Element4 : Inport  Port=5  PortName=wait_to_send  Element=signal
  In Bus Element6 : Inport  Port=5  PortName=wait_to_send  Element=signal
  In Bus Element5 : Inport  Port=5  PortName=wait_to_send  Element=package
  In Bus Element7 : Inport  Port=5  PortName=wait_to_send  Element=package
  Add_to_Send_Buffer : MATLAB Function  TreatAsAtomicUnit=on  SystemSampleTime=10/f
  Bus Creator : BusCreator  Inputs=4
  Bus Creator1 : BusCreator  Inputs=4
  Bus Creator2 : BusCreator  Inputs=4
  Bus Creator3 : BusCreator  Inputs=2
  Bus Creator4 : BusCreator  Inputs=3
  Data Store Memory : DataStoreMemory  DataStoreName=De_2  ReadBeforeWriteMsg=warning  WriteAfterWriteMsg=warning  WriteAfterReadMsg=warning  ShowAdditionalParam=off  OutDataTypeStr=double  Dimensions=1
  Data Store Memory1 : DataStoreMemory  DataStoreName=Recv_Buffer  ReadBeforeWriteMsg=warning  WriteAfterWriteMsg=warning  WriteAfterReadMsg=warning  InitialValue=zeros(20,7)  VectorParams1D=off  ShowAdditionalParam=off  OutDataTypeStr=double  Dimensions=[20,7]
  Data Store Memory10 : DataStoreMemory  DataStoreName=T_send_2  ReadBeforeWriteMsg=warning  WriteAfterWriteMsg=warning  WriteAfterReadMsg=warning  ShowAdditionalParam=off  OutDataTypeStr=double  Dimensions=1
  Data Store Memory11 : DataStoreMemory  DataStoreName=T_recv_2  ReadBeforeWriteMsg=warning  WriteAfterWriteMsg=warning  WriteAfterReadMsg=warning  ShowAdditionalParam=off  OutDataTypeStr=double  Dimensions=1
  Data Store Memory12 : DataStoreMemory  DataStoreName=Address  ReadBeforeWriteMsg=warning  WriteAfterWriteMsg=warning  WriteAfterReadMsg=warning  ShowAdditionalParam=off  OutDataTypeStr=double  Dimensions=1
  Data Store Memory13 : DataStoreMemory  DataStoreName=Address_1  ReadBeforeWriteMsg=warning  WriteAfterWriteMsg=warning  WriteAfterReadMsg=warning  ShowAdditionalParam=off  OutDataTypeStr=double  Dimensions=1
  Data Store Memory14 : DataStoreMemory  DataStoreName=Address_2  ReadBeforeWriteMsg=warning  WriteAfterWriteMsg=warning  WriteAfterReadMsg=warning  ShowAdditionalParam=off  OutDataTypeStr=double  Dimensions=1
  Data Store Memory15 : DataStoreMemory  DataStoreName=Handshake_1  ReadBeforeWriteMsg=warning  WriteAfterWriteMsg=warning  WriteAfterReadMsg=warning  InitialValue=false  ShowAdditionalParam=off  OutDataTypeStr=boolean
  Data Store Memory16 : DataStoreMemory  DataStoreName=Handshake_2  ReadBeforeWriteMsg=warning  WriteAfterWriteMsg=warning  WriteAfterReadMsg=warning  InitialValue=false  ShowAdditionalParam=off  OutDataTypeStr=boolean
  Data Store Memory2 : DataStoreMemory  DataStoreName=Send_Buffer_2  ReadBeforeWriteMsg=warning  WriteAfterWriteMsg=warning  WriteAfterReadMsg=warning  InitialValue=[101, 102, zeros(1,98)]  VectorParams1D=off  ShowAdditionalParam=off  OutDataTypeStr=double  Dimensions=[1,100]
  Data Store Memory3 : DataStoreMemory  DataStoreName=De_sum_1  ReadBeforeWriteMsg=warning  WriteAfterWriteMsg=warning  WriteAfterReadMsg=warning  ShowAdditionalParam=off  OutDataTypeStr=double  Dimensions=1
  Data Store Memory4 : DataStoreMemory  DataStoreName=De_sum_2  ReadBeforeWriteMsg=warning  WriteAfterWriteMsg=warning  WriteAfterReadMsg=warning  ShowAdditionalParam=off  OutDataTypeStr=double  Dimensions=1
  Data Store Memory5 : DataStoreMemory  DataStoreName=Send_Buffer_1  ReadBeforeWriteMsg=warning  WriteAfterWriteMsg=warning  WriteAfterReadMsg=warning  InitialValue=[101, 102, zeros(1,98)]  VectorParams1D=off  ShowAdditionalParam=off  OutDataTypeStr=double  Dimensions=[1,100]
  Data Store Memory6 : DataStoreMemory  DataStoreName=Filter  ReadBeforeWriteMsg=warning  WriteAfterWriteMsg=warning  WriteAfterReadMsg=warning  InitialValue=zeros(20,7)  VectorParams1D=off  ShowAdditionalParam=off  OutDataTypeStr=double  Dimensions=[20,7]
  Data Store Memory7 : DataStoreMemory  DataStoreName=De_1  ReadBeforeWriteMsg=warning  WriteAfterWriteMsg=warning  WriteAfterReadMsg=warning  ShowAdditionalParam=off  OutDataTypeStr=double  Dimensions=1
  Data Store Memory8 : DataStoreMemory  DataStoreName=T_send_1  ReadBeforeWriteMsg=warning  WriteAfterWriteMsg=warning  WriteAfterReadMsg=warning  ShowAdditionalParam=off  OutDataTypeStr=double  Dimensions=1
  Data Store Memory9 : DataStoreMemory  DataStoreName=T_recv_1  ReadBeforeWriteMsg=warning  WriteAfterWriteMsg=warning  WriteAfterReadMsg=warning  ShowAdditionalParam=off  OutDataTypeStr=double  Dimensions=1
  Data Store Read : DataStoreRead  DataStoreName=Send_Buffer_1
  Data Store Read1 : DataStoreRead  DataStoreName=Address
  Data Store Read10 : DataStoreRead  DataStoreName=De_sum_2
  Data Store Read11 : DataStoreRead  DataStoreName=De_sum_1
  Data Store Read12 : DataStoreRead  DataStoreName=T_send_2
  Data Store Read13 : DataStoreRead  DataStoreName=T_send_1
  Data Store Read14 : DataStoreRead  DataStoreName=T_recv_1
  Data Store Read15 : DataStoreRead  DataStoreName=T_recv_2
  Data Store Read16 : DataStoreRead  DataStoreName=De_2
  Data Store Read2 : DataStoreRead  DataStoreName=Filter
  Data Store Read3 : DataStoreRead  DataStoreName=Address_1
  Data Store Read4 : DataStoreRead  DataStoreName=Address_2
  Data Store Read5 : DataStoreRead  DataStoreName=Handshake_1
  Data Store Read6 : DataStoreRead  DataStoreName=Handshake_2
  Data Store Read7 : DataStoreRead  DataStoreName=Recv_Buffer
  Data Store Read8 : DataStoreRead  DataStoreName=Send_Buffer_2
  Data Store Read9 : DataStoreRead  DataStoreName=De_1
  Data Store Write : DataStoreWrite  DataStoreName=Address
  Delay1 : Delay  DelayLength=1
  Delay2 : Delay  DelayLength=1
  Display{,1..4,8..11,13} (10 alike) : Display
  Global_Var_Length : MATLAB Function  TreatAsAtomicUnit=on
  Memory2 : Memory  InitialCondition=false
  Recv_1 : MATLAB Function  TreatAsAtomicUnit=on  SystemSampleTime=10/f
  Recv_2 : MATLAB Function  TreatAsAtomicUnit=on  SystemSampleTime=10/f
  Scope : Scope
  Send_Telegram : Subsystem
  Send_to_Host : MATLAB Function  TreatAsAtomicUnit=on  SystemSampleTime=10/f
  Status : Stateflow chart  TreatAsAtomicUnit=on
  Time : Clock
      settings: Decimation=f
  Out Bus Element : Outport  PortName=Tx_1  Element=signal
  Out Bus Element1 : Outport  PortName=Tx_1  Element=data
  Out Bus Element2 : Outport  Port=2  PortName=Tx_2  Element=signal
  Out Bus Element3 : Outport  Port=2  PortName=Tx_2  Element=data
  status : Outport  Port=3
  send_done : Outport  Port=4
  Out Bus Element4 : Outport  Port=5  PortName=Recv  Element=signal
  Out Bus Element5 : Outport  Port=5  PortName=Recv  Element=package
  wires:
  ErrorSignal/1 -> Status/1(Error_Signal)
  Status/1(status) -> [status], status/1
  In Bus Element1/1 -> Recv_1/7(Rx_1_data)
  In Bus Element/1 -> Recv_1/6(Rx_1_signal)
  [status] -> Delay1/1
  Time/1 -> [clock]
  [clock] -> Recv_1/2(clock)
  Send_to_Host/1(signal) -> Out Bus Element4/1, Memory2/1
  address/1 -> Data Store Write/1
  Global_Var_Length/1(len_Send_Buffer_1) -> [len_Send_Buffer_1]
  Global_Var_Length/2(len_Send_Buffer_2) -> [len_Send_Buffer_2]
  Global_Var_Length/3(len_Recv_Buffer) -> [len_Recv_Buffer]
  Global_Var_Length/4(len_Filter) -> [len_Filter]
  [len_Send_Buffer_1] -> Recv_1/3(lenS_1)
  [len_Send_Buffer_2] -> Recv_1/4(lenS_2)
  [len_Recv_Buffer] -> Recv_1/5(lenR)
  In Bus Element2/1 -> Recv_2/6(Rx_2_signal)
  In Bus Element3/1 -> Recv_2/7(Rx_2_data)
  [status] -> Delay2/1
  [len_Recv_Buffer] -> Recv_2/5(lenR)
  [len_Send_Buffer_1] -> Recv_2/3(lenS_1)
  [clock] -> Recv_2/2(clock)
  [len_Send_Buffer_2] -> Recv_2/4(lenS_2)
  Delay1/1 -> Recv_1/1(status)
  Delay2/1 -> Recv_2/1(status)
  Recv_1/1(recv_signal_1) -> Status/2(recv_signal_1)
  Recv_1/2(recv_package_1) -> Status/3(recv_data_1)
  Recv_2/1(recv_signal_2) -> Status/4(recv_signal_2)
  Recv_2/2(recv_package_2) -> Status/5(recv_data_2)
  [len_Recv_Buffer] -> Send_to_Host/1(lenR)
  [len_Filter] -> Send_to_Host/2(lenF)
  [len_Send_Buffer_1] -> Add_to_Send_Buffer/2(lenS_1)
  [len_Send_Buffer_2] -> Add_to_Send_Buffer/3(lenS_2)
  In Bus Element4/1 -> Add_to_Send_Buffer/4(to_send_signal)
  In Bus Element5/1 -> Add_to_Send_Buffer/5(to_send_package)
  [status] -> Add_to_Send_Buffer/1(status)
  Memory2/1 -> Send_to_Host/3(signal_old)
  Bus Creator/1 -> Display/1
  [len_Send_Buffer_1] -> Bus Creator/1
  [len_Send_Buffer_2] -> Bus Creator/2
  [len_Recv_Buffer] -> Bus Creator/3
  [len_Filter] -> Bus Creator/4
  Data Store Read/1 -> Display1/1
  Data Store Read2/1 -> Display3/1
  Data Store Read8/1 -> Display8/1
  Data Store Read7/1 -> Display9/1
  Data Store Read13/1 -> Scope/1, Bus Creator1/1
  Data Store Read14/1 -> Bus Creator1/2
  Data Store Read11/1 -> Bus Creator1/4
  Data Store Read9/1 -> Bus Creator1/3
  Bus Creator1/1 -> Display10/1
  Data Store Read12/1 -> Bus Creator2/1
  Data Store Read15/1 -> Bus Creator2/2
  Bus Creator2/1 -> Display11/1
  Data Store Read16/1 -> Bus Creator2/3
  Data Store Read10/1 -> Bus Creator2/4
  [status] -> Display13/1
  Send_to_Host/2(package) -> Out Bus Element5/1
  Data Store Read5/1 -> Bus Creator3/1
  Data Store Read6/1 -> Bus Creator3/2
  Data Store Read4/1 -> Bus Creator4/3
  Data Store Read1/1 -> Bus Creator4/2
  Data Store Read3/1 -> Bus Creator4/1
  Bus Creator3/1 -> Display2/1
  Bus Creator4/1 -> Display4/1
  [status] -> Send_Telegram/1(status)
  [clock] -> Send_Telegram/2(clock)
  [len_Send_Buffer_1] -> Send_Telegram/3(lenS_1)
  [len_Send_Buffer_2] -> Send_Telegram/4(lenS_2)
  Send_Telegram/3(Tx_2_signal) -> Out Bus Element2/1
  Send_Telegram/4(Tx_2_data) -> Out Bus Element3/1
  Send_Telegram/2(Tx_1_data) -> Out Bus Element1/1
  Send_Telegram/1(Tx_1_signal) -> Out Bus Element/1
  Send_Telegram/5(send_done) -> send_done/1
  In Bus Element6/1 -> Send_Telegram/5(wait2send_sgn)
  In Bus Element7/1 -> Send_Telegram/6(wait2send_pkg)

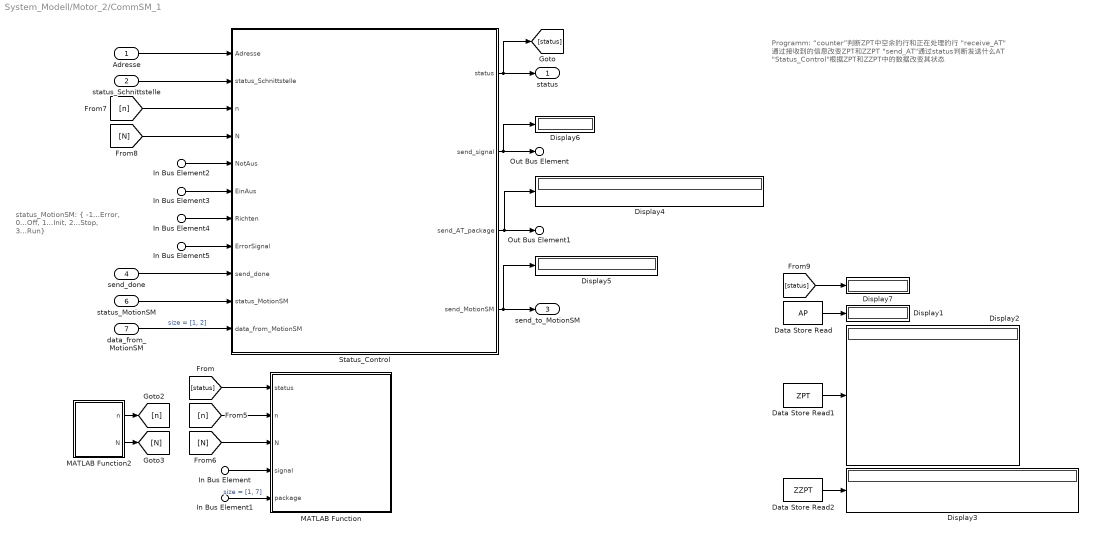
== system System_Modell/Motor_2/CommSM_1 ==
  note: Programm:
      | “counter”判断ZPT中空余的行和正在处理的行
      | "receive_AT" 通过接收到的信息改变ZPT和ZZPT
      | "send_AT"通过status判断发送什么AT
      | "Status_Control"根据ZPT和ZZPT中的数据改变其状态
  note: status_MotionSM: {
      | -1...Error,
      | 0...Off,
      | 1...Init,
      | 2...Stop,
      | 3...Run}
  Adresse : Inport  OutDataTypeStr=double  PortDimensions=1
  status_Schnittstelle : Inport  Port=2  OutDataTypeStr=double  PortDimensions=1
  In Bus Element2 : Inport  Port=3  PortName=Control  Element=NotAus
  In Bus Element3 : Inport  Port=3  PortName=Control  Element=EinAus
  In Bus Element4 : Inport  Port=3  PortName=Control  Element=Richten
  In Bus Element5 : Inport  Port=3  PortName=Control  Element=ErrorSignal
  send_done : Inport  Port=4
  In Bus Element : Inport  Port=5  PortName=Recv  Element=signal
  In Bus Element1 : Inport  Port=5  PortName=Recv  Element=package
  status_MotionSM : Inport  Port=6  OutDataTypeStr=double  PortDimensions=1
  data_from_MotionSM : Inport  Port=7  OutDataTypeStr=double  PortDimensions=2
  Data Store Read : DataStoreRead  DataStoreName=AP
  Data Store Read1 : DataStoreRead  DataStoreName=ZPT
  Data Store Read2 : DataStoreRead  DataStoreName=ZZPT
  Display{1..7} (7 alike) : Display
  MATLAB Function : MATLAB Function  TreatAsAtomicUnit=on
  MATLAB Function2 : MATLAB Function  TreatAsAtomicUnit=on
  Status_Control : Stateflow chart  TreatAsAtomicUnit=on
  status : Outport  OutDataTypeStr=double  PortDimensions=1
  Out Bus Element : Outport  Port=2  PortName=data_to_send  Element=signal
  Out Bus Element1 : Outport  Port=2  PortName=data_to_send  Element=package
  send_to_MotionSM : Outport  Port=3
  wires:
  In Bus Element2/1 -> Status_Control/5(NotAus)
  In Bus Element3/1 -> Status_Control/6(EinAus)
  In Bus Element4/1 -> Status_Control/7(Richten)
  In Bus Element5/1 -> Status_Control/8(ErrorSignal)
  status_Schnittstelle/1 -> Status_Control/2(status_Schnittstelle)
  In Bus Element/1 -> MATLAB Function/4(signal)
  In Bus Element1/1 -> MATLAB Function/5(package)  "size = [1, 7]"
  data_from_MotionSM/1 -> Status_Control/11(data_from_MotionSM)  "size = [1, 2]"
  status_MotionSM/1 -> Status_Control/10(status_MotionSM)
  Adresse/1 -> Status_Control/1(Adresse)
  Status_Control/1(status) -> [status], status/1
  Status_Control/3(send_AT_package) -> Out Bus Element1/1, Display4/1
  Status_Control/4(send_MotionSM) -> send_to_MotionSM/1, Display5/1
  Status_Control/2(send_signal) -> Out Bus Element/1, Display6/1
  Data Store Read/1 -> Display1/1
  Data Store Read1/1 -> Display2/1
  Data Store Read2/1 -> Display3/1
  [status] -> MATLAB Function/1(status)
  MATLAB Function2/1(n) -> [n]
  MATLAB Function2/2(N) -> [N]
  [N] -> MATLAB Function/3(N)
  [n] -> MATLAB Function/2(n)
  [n] -> Status_Control/3(n)
  [N] -> Status_Control/4(N)
  [status] -> Display7/1
  send_done/1 -> Status_Control/9(send_done)

== system System_Modell/Motor_2/MotionSM_1 ==
  note: parameter = [delta_T, a_max, v_max, s0]
  In Bus Element : Inport  PortName=Control  Element=NotAus
  In Bus Element1 : Inport  PortName=Control  Element=EinAus
  In Bus Element2 : Inport  PortName=Control  Element=Richten
  In Bus Element3 : Inport  PortName=Control  Element=ErrorSignal
  data_received : Inport  Port=2  OutDataTypeStr=double  PortDimensions=2
  delta_T : Inport  Port=3
  Bus Creator : BusCreator  Inputs=3
  Chart : Stateflow chart  TreatAsAtomicUnit=on
  Data Store Read : DataStoreRead  DataStoreName=AP
  Delay : Delay  DelayLength=1
  Delay1 : Delay  DelayLength=1
  Display{1..2,4..7} (6 alike) : Display
  MATLAB Function : MATLAB Function  TreatAsAtomicUnit=on
  Motor : Subsystem
  status : Outport
  data_to_send : Outport  Port=2  OutDataTypeStr=double  PortDimensions=2
  Out Bus Element : Outport  Port=3  PortName=Par  Element=a
  Out Bus Element1 : Outport  Port=3  PortName=Par  Element=v
  Out Bus Element2 : Outport  Port=3  PortName=Par  Element=s
  Out Bus Element3 : Outport  Port=3  PortName=Par  Element=AP
  wires:
  Chart/1(status) -> Motor/1(auto_control), Delay/1, Display1/1, status/1
  In Bus Element1/1 -> Chart/2(EinAus)
  In Bus Element/1 -> Chart/1(NotAus)
  In Bus Element2/1 -> Chart/3(Richten)
  In Bus Element3/1 -> Chart/4(ErrorSignal)
  Motor/1(status_Motor) -> Display4/1, Delay1/1
  data_received/1 -> MATLAB Function/2(data_received)
  Delay1/1 -> Chart/6(Motor_status)
  MATLAB Function/1(excute_signal) -> Display6/1, Chart/5(excute_signal)
  MATLAB Function/2(message_to_send) -> data_to_send/1, Display7/1  "size = [1, 2]"
  delta_T/1 -> Chart/7(delta_T)
  Motor/2(a) -> Bus Creator/3, Out Bus Element/1
  Motor/3(v) -> Bus Creator/2, Out Bus Element1/1
  Motor/4(s) -> Bus Creator/1, Out Bus Element2/1
  Chart/2(parameter) -> Motor/2(parameter), Display5/1
  Delay/1 -> MATLAB Function/1(status)
  Data Store Read/1 -> Out Bus Element3/1
  Bus Creator/1 -> Display2/1
